simulink model "a_4_model_"  (R2020a)
settings: Solver=VariableStepAuto  StartTime=0.0  StopTime=10.0  RelTol=1e-3
values from neighbouring files (symbols this model uses):
  altitude = alt    [trim_f16_modified.m]
  model = struct()    [find_f16_dynamics.m]
  velocity = vel    [trim_f16_modified.m]
settings Model: Creator=adewindt  LastModifiedBy=adewindt

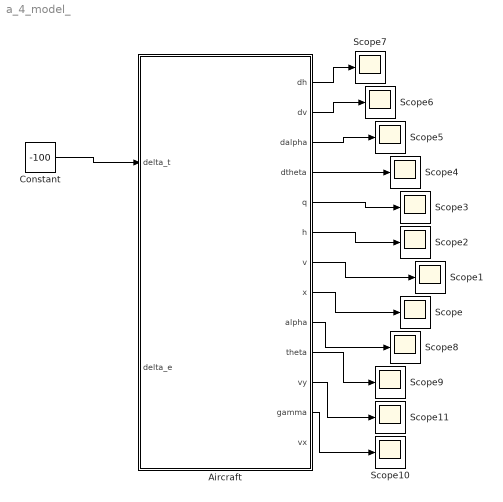
== system a_4_model_ ==
  Aircraft : Subsystem
  Constant : Constant  Value=-100
  Scope{,1..11} (12 alike) : Scope
  wires:
  Aircraft/8(x) -> Scope/1
  Aircraft/7(v) -> Scope1/1
  Aircraft/6(h) -> Scope2/1
  Aircraft/5(q) -> Scope3/1
  Aircraft/4(dtheta) -> Scope4/1
  Aircraft/3(dalpha) -> Scope5/1
  Aircraft/2(dv) -> Scope6/1
  Aircraft/1(dh) -> Scope7/1
  Aircraft/9(alpha) -> Scope8/1
  Aircraft/10(theta) -> Scope9/1
  Aircraft/12(gamma) -> Scope10/1
  Aircraft/11(vy) -> Scope11/1
  Constant/1 -> Aircraft/1(delta_t)

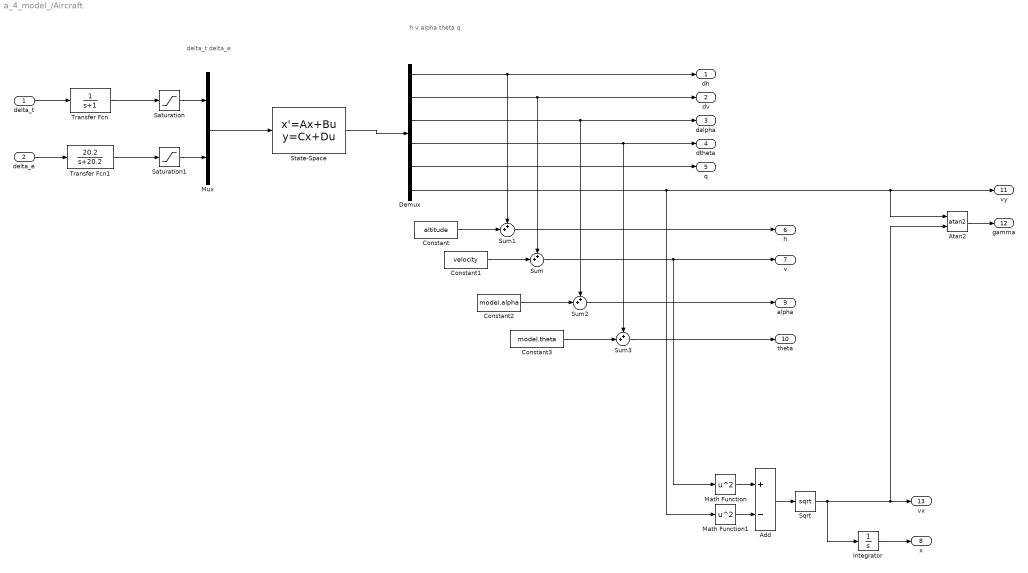
== system a_4_model_/Aircraft ==
  note: delta_t delta_e
  note: h v alpha theta q
  delta_t : Inport
  delta_e : Inport  Port=2
  Add : Sum  Inputs=+-
  Atan2 : Trigonometry  Operator=atan2
  Constant : Constant  Value=altitude
  Constant1 : Constant  Value=velocity
  Constant2 : Constant  Value=model.alpha
  Constant3 : Constant  Value=model.theta
  Demux : Demux  Outputs=6
  Integrator : Integrator  InitialCondition=-41162
  Math Function : Math  Operator=square  SaturateOnIntegerOverflow=on
  Math Function1 : Math  Operator=square  SaturateOnIntegerOverflow=on
  Mux : Mux  Inputs=2
  Saturation : Saturate  UpperLimit=19000-model.thrust  LowerLimit=1000-model.thrust
  Saturation1 : Saturate  UpperLimit=25-model.delta_e  LowerLimit=-25-model.delta_e
  Sqrt : Sqrt  SaturateOnIntegerOverflow=on
  State-Space : StateSpace  A=model.ss_landing.A  B=model.ss_landing.B  C=model.ss_landing.C  D=model.ss_landing.D  InitialCondition=0
  Sum{,1..3} (4 alike) : Sum  Inputs=++|
  Transfer Fcn : TransferFcn  Denominator=[1 1]
  Transfer Fcn1 : TransferFcn  Numerator=[20.2]  Denominator=[1 20.2]
  dh : Outport
  dv : Outport  Port=2
  dalpha : Outport  Port=3
  dtheta : Outport  Port=4
  q : Outport  Port=5
  h : Outport  Port=6
  v : Outport  Port=7
  x : Outport  Port=8
  alpha : Outport  Port=9
  theta : Outport  Port=10
  vy : Outport  Port=11
  gamma : Outport  Port=12
  vx : Outport  Port=13
  wires:
  Mux/1 -> State-Space/1
  delta_t/1 -> Transfer Fcn/1
  delta_e/1 -> Transfer Fcn1/1
  State-Space/1 -> Demux/1
  Transfer Fcn/1 -> Saturation/1
  Transfer Fcn1/1 -> Saturation1/1
  Saturation1/1 -> Mux/2
  Demux/5 -> q/1
  Demux/1 -> Sum1/1, dh/1
  Saturation/1 -> Mux/1
  Demux/3 -> Sum2/1, dalpha/1
  Demux/2 -> Sum/1, dv/1
  Constant2/1 -> Sum2/2
  Constant1/1 -> Sum/2
  Constant/1 -> Sum1/2
  Constant3/1 -> Sum3/2
  Demux/4 -> Sum3/1, dtheta/1
  Sum1/1 -> h/1
  Sum/1 -> v/1, Math Function/1
  Sum3/1 -> theta/1
  Sum2/1 -> alpha/1
  Integrator/1 -> x/1
  Demux/6 -> vy/1, Atan2/1, Math Function1/1
  Atan2/1 -> gamma/1
  Math Function/1 -> Add/1
  Math Function1/1 -> Add/2
  Add/1 -> Sqrt/1
  Sqrt/1 -> Integrator/1, Atan2/2, vx/1
